simulink model "SVPWM"  (R2023b)
settings: Solver=FixedStepAuto  StartTime=0.0  StopTime=10.0  FixedStep=0.005  RelTol=1e-3
libraries: mcbcontrolslib x2, spsSawtoothGeneratorLib x1
settings Model: Creator=LZQ  LastModifiedBy=LZQ

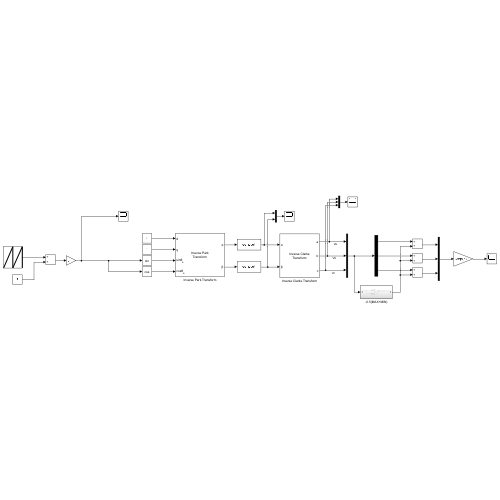
[thumbnail: Simulink's stored preview of the top-level diagram]
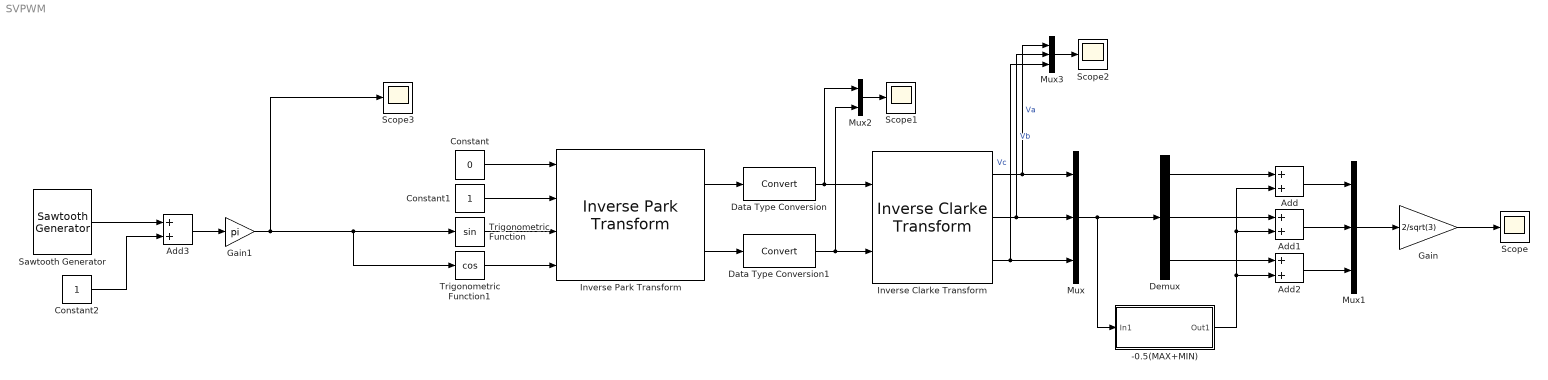
== system SVPWM ==
  -0.5(MAX+MIN) : Subsystem
  Add{,1..3} (4 alike) : Sum
  Constant : Constant  Value=0
  Constant1 : Constant
  Constant2 : Constant
  Data Type Conversion : DataTypeConversion  SaturateOnIntegerOverflow=off  RndMeth=Floor
  Data Type Conversion1 : DataTypeConversion  SaturateOnIntegerOverflow=off  RndMeth=Floor
  Demux : Demux  Outputs=3
  Gain : Gain  Gain=2/sqrt(3)
  Gain1 : Gain  Gain=pi
  Inverse Clarke Transform : mcbcontrolslib/Inverse Clarke Transform  PhaseInput=Two inputs  EnPowerInv=off
      settings: LibrarySourceBlock=mcblib/Controls/Math Transforms/Inverse Clarke Transform
  Inverse Park Transform : mcbcontrolslib/Inverse Park Transform  PhaseInput=Two inputs  AxisAlignment=D-axis  ThetaInput=Sine and Cosine electrical position  AngleInput=Per-unit  N_points=1024
      settings: LibrarySourceBlock=mcblib/Controls/Math Transforms/Inverse Park Transform
  Mux : Mux  Inputs=3
  Mux1 : Mux  Inputs=3
  Mux2 : Mux  Inputs=2
  Mux3 : Mux  Inputs=3
  Sawtooth Generator : spsSawtoothGeneratorLib/Sawtooth Generator  Freq=1  Phase=360  Ts=0
  Scope{,1..3} (4 alike) : Scope
  Trigonometric Function : Trigonometry
  Trigonometric Function1 : Trigonometry  Operator=cos
  wires:
  Constant/1 -> Inverse Park Transform/1
  Constant1/1 -> Inverse Park Transform/2
  Inverse Park Transform/1 -> Data Type Conversion/1
  Inverse Park Transform/2 -> Data Type Conversion1/1
  Data Type Conversion/1 -> Mux2/1, Inverse Clarke Transform/1
  Data Type Conversion1/1 -> Mux2/2, Inverse Clarke Transform/2
  Inverse Clarke Transform/1 -> Mux3/1, Mux/1  "Va"
  Inverse Clarke Transform/2 -> Mux3/2, Mux/2  "Vb"
  Inverse Clarke Transform/3 -> Mux3/3, Mux/3  "Vc"
  Demux/1 -> Add/1
  Demux/2 -> Add1/1
  Demux/3 -> Add2/1
  -0.5(MAX+MIN)/1(Out1) -> Add2/2, Add1/2, Add/2
  Add/1 -> Mux1/1
  Add1/1 -> Mux1/2
  Add2/1 -> Mux1/3
  Gain/1 -> Scope/1
  Gain1/1 -> Scope3/1, Trigonometric Function1/1, Trigonometric Function/1
  Mux/1 -> -0.5(MAX+MIN)/1(In1), Demux/1
  Mux1/1 -> Gain/1
  Mux2/1 -> Scope1/1
  Trigonometric Function/1 -> Inverse Park Transform/3
  Trigonometric Function1/1 -> Inverse Park Transform/4
  Constant2/1 -> Add3/2
  Sawtooth Generator/1 -> Add3/1
  Add3/1 -> Gain1/1
  Mux3/1 -> Scope2/1

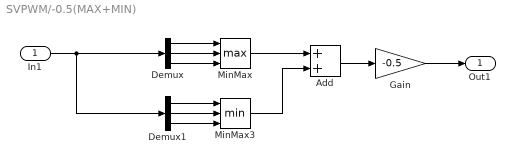
== system SVPWM/-0.5(MAX+MIN) ==
  In1 : Inport
  Add : Sum
  Demux : Demux  Outputs=3
  Demux1 : Demux  Outputs=3
  Gain : Gain  Gain=-0.5
  MinMax : MinMax  Function=max  Inputs=3
  MinMax3 : MinMax  Inputs=3
  Out1 : Outport
  wires:
  In1/1 -> Demux1/1, Demux/1
  Demux/1 -> MinMax/1
  Demux/2 -> MinMax/2
  Demux/3 -> MinMax/3
  Demux1/1 -> MinMax3/1
  Demux1/2 -> MinMax3/2
  Demux1/3 -> MinMax3/3
  MinMax/1 -> Add/1
  MinMax3/1 -> Add/2
  Add/1 -> Gain/1
  Gain/1 -> Out1/1
